simulink model "test2"  (R2016b)
settings: Solver=VariableStepAuto  StartTime=0.0  StopTime=10.0  RelTol=1e-3
values from neighbouring files (symbols this model uses):
  bore_max = 20e-6    (= 2e-05)    [Active_Body_Control_param_stud.m]
  delta_y_s = 0.005    [Active_Body_Control_param_stud.m]
  s_max_va = 0.020    (= 0.02)    [Active_Body_Control_param_stud.m]
settings Model: Creator=ti.unbehaun  LastModifiedBy=ti.unbehaun

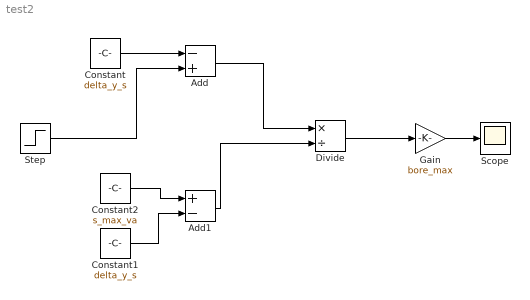
== system test2 ==
  Add : Sum  Inputs=-+
  Add1 : Sum  Inputs=+-
  Constant : Constant  Value=delta_y_s
  Constant1 : Constant  Value=delta_y_s
  Constant2 : Constant  Value=s_max_va
  Divide : Product  Inputs=*/
  Gain : Gain  Gain=bore_max
  Scope : Scope
  Step : Step  Time=5  After=0.015  SampleTime=0
  wires:
  Step/1 -> Add/2
  Constant/1 -> Add/1
  Add/1 -> Divide/1
  Add1/1 -> Divide/2
  Constant1/1 -> Add1/2
  Constant2/1 -> Add1/1
  Divide/1 -> Gain/1
  Gain/1 -> Scope/1
